simulink model "transmitancja"  (R2020a)
settings: Solver=VariableStepAuto  StartTime=0.0  StopTime=10.0  RelTol=1e-3
values from neighbouring files (symbols this model uses):
  dTkz0 = 0    [Skrypt.m]    (also in proj.m)
  dTzew0 = 0    [Skrypt.m]    (also in proj.m)
  G11a = Cv2*xp0    (= 180000000)    [proj.m]
  G11b = (xp0+K0+Ks2)*xp0    (= 8228571.42857)    [proj.m]
  G12a = Ks1*Cv1    (= 27000000)    [proj.m]
  G12b = Ks1*(xp0+Ks2+K0)+K0*Ks2    (= 2057142.85714)    [proj.m]
  G21a = (K0+xp0)*xp0    (= 7200000)    [proj.m]
  G22a = Cv1*Ks2    (= 46285714.2857)    [proj.m]
  G22b = Ks2*(xp0+Ks1+K0)+K0*Ks1+xp0*Ks1    (= 3085714.28571)    [proj.m]
  M1 = Cv1*Cv2    (= 8100000000)    [proj.m]
  M2 = (Cv1*Ks2+Cv1*K0+Cv1*xp0+K0*Cv2+Ks1*Cv2+xp0*Cv2)    (= 721285714.286)    [proj.m]
  M3 = (xp0^2+xp0*Ks2+xp0*Ks1+K0*Ks1+Ks1*Ks2+K0*xp0+K0*Ks2)    (= 10285714.2857)    [proj.m]
  steptime = 50    [proj.m]
  Tw10 = (((xp0*Tkz1 + Ks1*Tzew0)*(K0+xp0+Ks2))+ Ks2*Tzew0*K0)/((xp0+Ks1+K0)*(K0+xp0+Ks2)-(K0^2+xp0*K0))    [Skrypt.m]    (also in proj.m)
  Tw20 = (Tw10*(K0+xp0) + Ks2*Tzew0)/(K0 + xp0 + Ks2)    (= 15)    [Skrypt.m]    (also in proj.m)
settings Model: Creator=pc  LastModifiedBy=pc

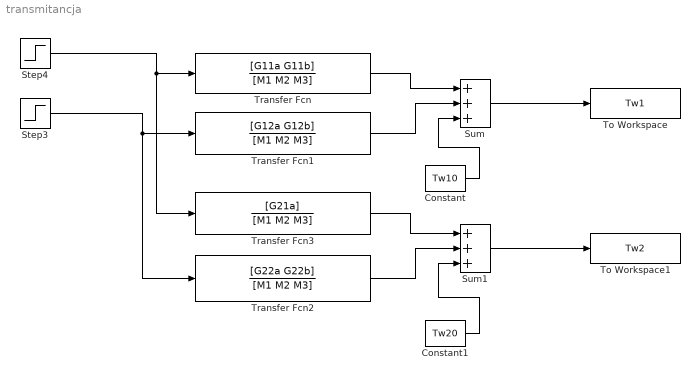
== system transmitancja ==
  Constant : Constant  Value=Tw10
  Constant1 : Constant  Value=Tw20
  Step3 : Step  Time=steptime  After=0+dTzew0  SampleTime=0
  Step4 : Step  Time=steptime  After=0+dTkz0  SampleTime=0
  Sum : Sum  Inputs=+++
  Sum1 : Sum  Inputs=+++
  To Workspace : ToWorkspace  VariableName=Tw1  SampleTime=-1
  To Workspace1 : ToWorkspace  VariableName=Tw2  SampleTime=-1
  Transfer Fcn : TransferFcn  Numerator=[G11a G11b]  Denominator=[M1 M2 M3]
  Transfer Fcn1 : TransferFcn  Numerator=[G12a G12b]  Denominator=[M1 M2 M3]
  Transfer Fcn2 : TransferFcn  Numerator=[G22a G22b]  Denominator=[M1 M2 M3]
  Transfer Fcn3 : TransferFcn  Numerator=[G21a]  Denominator=[M1 M2 M3]
  wires:
  Constant1/1 -> Sum1/3
  Constant/1 -> Sum/3
  Transfer Fcn3/1 -> Sum1/1
  Sum1/1 -> To Workspace1/1
  Sum/1 -> To Workspace/1
  Transfer Fcn1/1 -> Sum/2
  Transfer Fcn/1 -> Sum/1
  Transfer Fcn2/1 -> Sum1/2
  Step4/1 -> Transfer Fcn3/1, Transfer Fcn/1
  Step3/1 -> Transfer Fcn2/1, Transfer Fcn1/1
